simulink model "Test_FourMotor_PID_simcape_motor"  (R2025a)
settings: Solver=FixedStepAuto  StartTime=0.0  StopTime=2  FixedStep=50e-5  RelTol=1e-3
values from neighbouring files (symbols this model uses):
  Ki_id = 710.3004    [EMRAX348_DQData.m]    (also in Evolito_D500_DQData.m = 281.669634183)
  Ki_iq = 1.0615e3    (= 1061.5)    [EMRAX348_DQData.m]    (also in Evolito_D500_DQData.m = 420.937840785)
  Kp_id = 0.8779    [EMRAX348_DQData.m]    (also in Evolito_D500_DQData.m = 0.144107025607)
  Kp_iq = 1.0744    [EMRAX348_DQData.m]    (also in Evolito_D500_DQData.m = 0.144418307682)
  Ld = 52e-6    (= 5.2e-05)    [EMRAX348_DQData.m]    (also in Evolito_D500_DQData.m = 4e-05; pmsm_batt_testbench_data.m = 4e-05)
  Lq = 52e-6    (= 5.2e-05)    [EMRAX348_DQData.m]    (also in Evolito_D500_DQData.m = 4e-05; pmsm_batt_testbench_data.m = 4e-05)
  p = 10    [EMRAX348_DQData.m]    (also in Evolito_D500_DQData.m; pmsm_batt_testbench_data.m)
  psim = 0.06249    [EMRAX348_DQData.m]    (also in Evolito_D500_DQData.m = 0.045; pmsm_batt_testbench_data.m = 0.045)
undefined symbols (not defined in the file or in its folder): Limit, motorctrl, RPM
libraries: fl_lib x101, nesl_utility x37, eeDiscretePi x8, slpidlib x7, eeDqVoltageLimiter x4, eePmsmCurrentReferenceGen x4, eePmsmTorqueEstimator x4, ee_lib x4, batteryecm_lib x2, HEV_Battery_Lib x1, spspowerguiLib x1
(part 1 of 3)
settings Model: Creator=froshoo  LastModifiedBy=froshoo
settings DataIOCC: SaveOutput=off  SignalLogging=off  DSMLogging=off  SaveTime=off  ReturnWorkspaceOutputs=off
settings SimscapeCC: SimscapeLogType=all  SimscapeLogSimulationStatistics=on  SimscapeLogToSDI=on  SimscapeLogOpenViewer=on

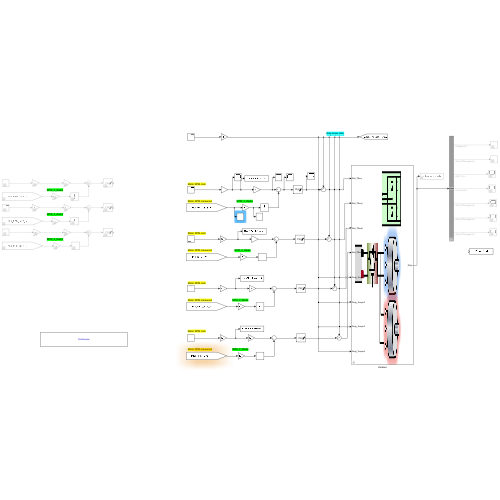
[thumbnail: Simulink's stored preview of the top-level diagram]
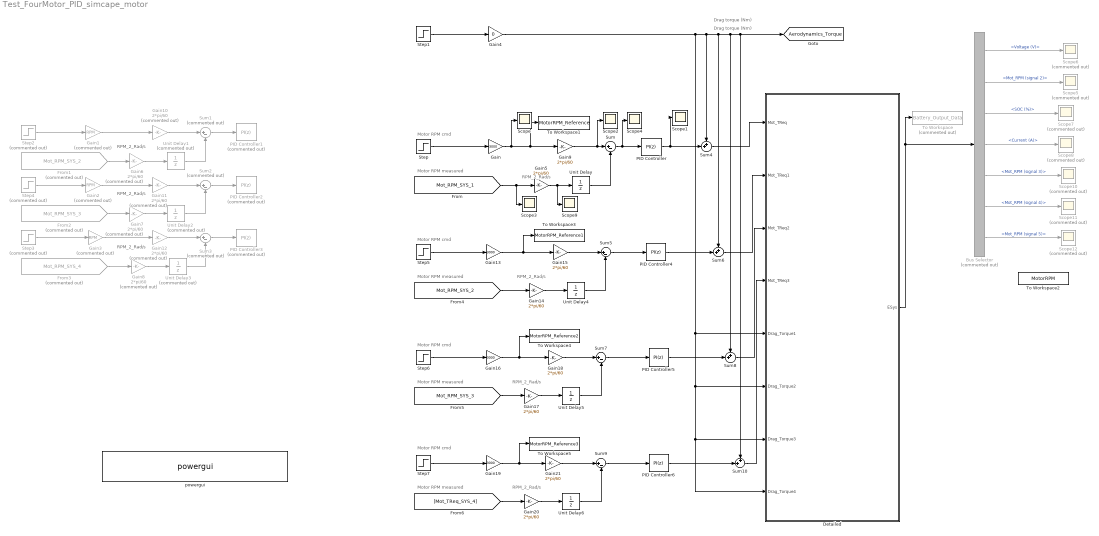
== system Test_FourMotor_PID_simcape_motor ==
  note: Motor RPM cmd
  note: Motor RPM measured
  note: RPM_2_Rad/s
  note: RPM_2_Rad/s
  note: RPM_2_Rad/s
  note: RPM_2_Rad/s
  note: Drag torque (Nm)
  note: Drag torque (Nm)
  note: RPM_2_Rad/s
  note: Motor RPM cmd
  note: Motor RPM measured
  note: Motor RPM measured
  note: RPM_2_Rad/s
  note: Motor RPM cmd
  note: Motor RPM cmd
  note: Motor RPM measured
  note: RPM_2_Rad/s
  Bus Selector : BusSelector  Commented=on  OutputSignals=Batt (signal 1).Voltage (V),Mot_RPM (signal 2),Batt (signal 1).SOC (%),Batt (signal 1).Current (A),Mot_RPM (signal 3),Mot_RPM (signal 4),Mot_RPM (signal 5)
  Detailed : Subsystem  mask{popup_batteryvariant=Cells}
      mask prompts: popup_batteryvariant "Battery Model"
      mask init:
      | set_param([gcb '/Battery'],'LabelModeActiveChoice',get_param(gcb,'popup_batteryvariant'));
      mask TypeOptions popup_batteryvariant: Predefined | Cells | Generic
      mask Display: image('HEV_Electrical_Detailed_IMAGE.jpg');
  From1 : From  Commented=on  GotoTag=Mot_RPM_SYS_2  TagVisibility=global
  From2 : From  Commented=on  GotoTag=Mot_RPM_SYS_3  TagVisibility=global
  From3 : From  Commented=on  GotoTag=Mot_RPM_SYS_4  TagVisibility=global
  Gain{,13,16,19} (4 alike) : Gain  Gain=3000
  Gain1 : Gain  Commented=on  Gain=RPM
  Gain{6..8,10..12} (6 alike) : Gain  Commented=on  Gain=2*pi/60
  Gain{5,9,14..15,17..18,20..21} (8 alike) : Gain  Gain=2*pi/60
  Gain2 : Gain  Commented=on  Gain=RPM
  Gain3 : Gain  Commented=on  Gain=RPM
  Gain4 : Gain  Gain=0
  PID Controller{,4..6} (4 alike) : slpidlib/PID Controller  Controller=PI  Form=Parallel  TimeDomain=Discrete-time  UseExternalTs=off  SampleTime=0.005  IntegratorMethod=Forward Euler  FilterMethod=Forward Euler  ControllerParametersSource=internal  P=0.4  I=0.5  UseKiTs=off  D=motorctrl.d  UseExternalDerivativeSource=off  N=motorctrl.n  UseFilter=on  TunerSelectOption=Transfer Function Based (PID Tuner App)  InitialConditionSource=internal  InitialConditionForIntegrator=0  InitialConditionForFilter=0  DifferentiatorICPrevScaledInput=0  ExternalReset=none  TrackingMode=off  Kt=1  LimitOutput=on  SatLimitsSource=internal  UpperSaturationLimit=800  LowerSaturationLimit=-800  LinearizeAsGain=on  AntiWindupMode=back-calculation  Kb=1  LimitIntegrator=off  UpperIntegratorSaturationLimit=inf  LowerIntegratorSaturationLimit=-inf  POutMin=[]  POutMax=[]  IOutMin=[]  IOutMax=[]  DOutMin=[]  DOutMax=[]  NOutMin=[]  NOutMax=[]  SumOutMin=[]  SumOutMax=[]  SaturationOutMin=[]  SaturationOutMax=[]  PParamMin=[]  PParamMax=[]  IParamMin=[]  IParamMax=[]  DParamMin=[]  DParamMax=[]  NParamMin=[]  NParamMax=[]  KbParamMin=[]  KbParamMax=[]  KtParamMin=[]  KtParamMax=[]  KbOutMin=[]  KbOutMax=[]  KtOutMin=[]  KtOutMax=[]  IntegratorOutMin=[]  IntegratorOutMax=[]  FilterOutMin=[]  FilterOutMax=[]  SumI1OutMin=[]  SumI1OutMax=[]  SumI2OutMin=[]  SumI2OutMax=[]  SumI3OutMin=[]  SumI3OutMax=[]  SumI4OutMin=[]  SumI4OutMax=[]  SumDOutMin=[]  SumDOutMax=[]  DifferentiatorOutMin=[]  DifferentiatorOutMax=[]  FilterDiffOutCoefMin=[]  FilterDiffOutCoefMax=[]  ReciprocalOutMin=[]  ReciprocalOutMax=[]  SumDenOutMin=[]  SumDenOutMax=[]  SumNumOutMin=[]  SumNumOutMax=[]  DivideOutMin=[]  DivideOutMax=[]  UdiffTsProdOutMin=[]  UdiffTsProdOutMax=[]  NTsProdOutMin=[]  NTsProdOutMax=[]  UintegralTsProdOutMin=[]  UintegralTsProdOutMax=[]  UngainTsProdOutMin=[]  UngainTsProdOutMax=[]  ClampingZeroOutDataTypeStr=Inherit: Inherit via back propagation  ClampingZeroOutMin=[]  ClampingZeroOutMax=[]  FilterDenConstantOutDataTypeStr=Inherit: Inherit via back propagation  FilterDenConstantOutMin=[]  FilterDenConstantOutMax=[]  PCopyOutDataTypeStr=Inherit: Inherit via back propagation  PCopyOutMin=[]  PCopyOutMax=[]  NCopyOutDataTypeStr=Inherit: Inherit via back propagation  NCopyOutMin=[]  NCopyOutMax=[]  IntegratorContinuousStateAttributes=''  IntegratorStateMustResolveToSignalObject=off  IntegratorRTWStateStorageClass=Auto  FilterContinuousStateAttributes=''  FilterStateMustResolveToSignalObject=off  FilterRTWStateStorageClass=Auto  ParallelPVariant=InternalParameters  IdealPVariant=Disabled  IVariant=InternalParameters  DVariant=Disabled  IntegratorVariant=Discrete  SatVariant=Enabled  AWVariant=BackCalculation  PCopyVariant=Disabled  TRVariant=Disabled  FdbkBlocksVariant=Forward  IdealPFdbkVariant=Disabled  SatFdbkVariant=Disabled  DerivativeFilterVariant=Disabled  NVariant=Disabled  NCopyVariant=Disabled_SignalSpec  FilterICVariant=Disabled  IntegratorICVariant=InternalICs  ExternalResetVariant=Disabled  TRSumVariant=Passthrough  SumFdbkVariant=Disabled  SumVariant=Sum_PI  TsampFilterVariant=InternalTs  TsampNgainVariant=Passthrough  TsampIntegralVariant=Disabled_SignalSpec  ExternalSaturationOutDataTypeStr=Inherit: Same as second input  DerivativeSourceVariant=Disabled  PreIntVariant=InternalPreInt
  PID Controller1 : slpidlib/PID Controller  Commented=on  Controller=PI  Form=Parallel  TimeDomain=Discrete-time  UseExternalTs=off  SampleTime=0.005  IntegratorMethod=Forward Euler  FilterMethod=Forward Euler  ControllerParametersSource=internal  P=motorctrl.p  I=motorctrl.i  UseKiTs=off  D=motorctrl.d  UseExternalDerivativeSource=off  N=motorctrl.n  UseFilter=on  TunerSelectOption=Transfer Function Based (PID Tuner App)  InitialConditionSource=internal  InitialConditionForIntegrator=0  InitialConditionForFilter=0  DifferentiatorICPrevScaledInput=0  ExternalReset=none  TrackingMode=off  Kt=1  LimitOutput=on  SatLimitsSource=internal  UpperSaturationLimit=Limit  LowerSaturationLimit=-Limit  LinearizeAsGain=on  AntiWindupMode=back-calculation  Kb=1  LimitIntegrator=off  UpperIntegratorSaturationLimit=inf  LowerIntegratorSaturationLimit=-inf  POutMin=[]  POutMax=[]  IOutMin=[]  IOutMax=[]  DOutMin=[]  DOutMax=[]  NOutMin=[]  NOutMax=[]  SumOutMin=[]  SumOutMax=[]  SaturationOutMin=[]  SaturationOutMax=[]  PParamMin=[]  PParamMax=[]  IParamMin=[]  IParamMax=[]  DParamMin=[]  DParamMax=[]  NParamMin=[]  NParamMax=[]  KbParamMin=[]  KbParamMax=[]  KtParamMin=[]  KtParamMax=[]  KbOutMin=[]  KbOutMax=[]  KtOutMin=[]  KtOutMax=[]  IntegratorOutMin=[]  IntegratorOutMax=[]  FilterOutMin=[]  FilterOutMax=[]  SumI1OutMin=[]  SumI1OutMax=[]  SumI2OutMin=[]  SumI2OutMax=[]  SumI3OutMin=[]  SumI3OutMax=[]  SumI4OutMin=[]  SumI4OutMax=[]  SumDOutMin=[]  SumDOutMax=[]  DifferentiatorOutMin=[]  DifferentiatorOutMax=[]  FilterDiffOutCoefMin=[]  FilterDiffOutCoefMax=[]  ReciprocalOutMin=[]  ReciprocalOutMax=[]  SumDenOutMin=[]  SumDenOutMax=[]  SumNumOutMin=[]  SumNumOutMax=[]  DivideOutMin=[]  DivideOutMax=[]  UdiffTsProdOutMin=[]  UdiffTsProdOutMax=[]  NTsProdOutMin=[]  NTsProdOutMax=[]  UintegralTsProdOutMin=[]  UintegralTsProdOutMax=[]  UngainTsProdOutMin=[]  UngainTsProdOutMax=[]  ClampingZeroOutDataTypeStr=Inherit: Inherit via back propagation  ClampingZeroOutMin=[]  ClampingZeroOutMax=[]  FilterDenConstantOutDataTypeStr=Inherit: Inherit via back propagation  FilterDenConstantOutMin=[]  FilterDenConstantOutMax=[]  PCopyOutDataTypeStr=Inherit: Inherit via back propagation  PCopyOutMin=[]  PCopyOutMax=[]  NCopyOutDataTypeStr=Inherit: Inherit via back propagation  NCopyOutMin=[]  NCopyOutMax=[]  IntegratorContinuousStateAttributes=''  IntegratorStateMustResolveToSignalObject=off  IntegratorRTWStateStorageClass=Auto  FilterContinuousStateAttributes=''  FilterStateMustResolveToSignalObject=off  FilterRTWStateStorageClass=Auto  ParallelPVariant=InternalParameters  IdealPVariant=Disabled  IVariant=InternalParameters  DVariant=Disabled  IntegratorVariant=Discrete  SatVariant=Enabled  AWVariant=BackCalculation  PCopyVariant=Disabled  TRVariant=Disabled  FdbkBlocksVariant=Forward  IdealPFdbkVariant=Disabled  SatFdbkVariant=Disabled  DerivativeFilterVariant=Disabled  NVariant=Disabled  NCopyVariant=Disabled_SignalSpec  FilterICVariant=Disabled  IntegratorICVariant=InternalICs  ExternalResetVariant=Disabled  TRSumVariant=Passthrough  SumFdbkVariant=Disabled  SumVariant=Sum_PI  TsampFilterVariant=InternalTs  TsampNgainVariant=Passthrough  TsampIntegralVariant=Disabled_SignalSpec  ExternalSaturationOutDataTypeStr=Inherit: Same as second input  DerivativeSourceVariant=Disabled  PreIntVariant=InternalPreInt
  PID Controller2 : slpidlib/PID Controller  Commented=on  Controller=PI  Form=Parallel  TimeDomain=Discrete-time  UseExternalTs=off  SampleTime=0.005  IntegratorMethod=Forward Euler  FilterMethod=Forward Euler  ControllerParametersSource=internal  P=motorctrl.p  I=motorctrl.i  UseKiTs=off  D=motorctrl.d  UseExternalDerivativeSource=off  N=motorctrl.n  UseFilter=on  TunerSelectOption=Transfer Function Based (PID Tuner App)  InitialConditionSource=internal  InitialConditionForIntegrator=0  InitialConditionForFilter=0  DifferentiatorICPrevScaledInput=0  ExternalReset=none  TrackingMode=off  Kt=1  LimitOutput=on  SatLimitsSource=internal  UpperSaturationLimit=Limit  LowerSaturationLimit=-Limit  LinearizeAsGain=on  AntiWindupMode=back-calculation  Kb=1  LimitIntegrator=off  UpperIntegratorSaturationLimit=inf  LowerIntegratorSaturationLimit=-inf  POutMin=[]  POutMax=[]  IOutMin=[]  IOutMax=[]  DOutMin=[]  DOutMax=[]  NOutMin=[]  NOutMax=[]  SumOutMin=[]  SumOutMax=[]  SaturationOutMin=[]  SaturationOutMax=[]  PParamMin=[]  PParamMax=[]  IParamMin=[]  IParamMax=[]  DParamMin=[]  DParamMax=[]  NParamMin=[]  NParamMax=[]  KbParamMin=[]  KbParamMax=[]  KtParamMin=[]  KtParamMax=[]  KbOutMin=[]  KbOutMax=[]  KtOutMin=[]  KtOutMax=[]  IntegratorOutMin=[]  IntegratorOutMax=[]  FilterOutMin=[]  FilterOutMax=[]  SumI1OutMin=[]  SumI1OutMax=[]  SumI2OutMin=[]  SumI2OutMax=[]  SumI3OutMin=[]  SumI3OutMax=[]  SumI4OutMin=[]  SumI4OutMax=[]  SumDOutMin=[]  SumDOutMax=[]  DifferentiatorOutMin=[]  DifferentiatorOutMax=[]  FilterDiffOutCoefMin=[]  FilterDiffOutCoefMax=[]  ReciprocalOutMin=[]  ReciprocalOutMax=[]  SumDenOutMin=[]  SumDenOutMax=[]  SumNumOutMin=[]  SumNumOutMax=[]  DivideOutMin=[]  DivideOutMax=[]  UdiffTsProdOutMin=[]  UdiffTsProdOutMax=[]  NTsProdOutMin=[]  NTsProdOutMax=[]  UintegralTsProdOutMin=[]  UintegralTsProdOutMax=[]  UngainTsProdOutMin=[]  UngainTsProdOutMax=[]  ClampingZeroOutDataTypeStr=Inherit: Inherit via back propagation  ClampingZeroOutMin=[]  ClampingZeroOutMax=[]  FilterDenConstantOutDataTypeStr=Inherit: Inherit via back propagation  FilterDenConstantOutMin=[]  FilterDenConstantOutMax=[]  PCopyOutDataTypeStr=Inherit: Inherit via back propagation  PCopyOutMin=[]  PCopyOutMax=[]  NCopyOutDataTypeStr=Inherit: Inherit via back propagation  NCopyOutMin=[]  NCopyOutMax=[]  IntegratorContinuousStateAttributes=''  IntegratorStateMustResolveToSignalObject=off  IntegratorRTWStateStorageClass=Auto  FilterContinuousStateAttributes=''  FilterStateMustResolveToSignalObject=off  FilterRTWStateStorageClass=Auto  ParallelPVariant=InternalParameters  IdealPVariant=Disabled  IVariant=InternalParameters  DVariant=Disabled  IntegratorVariant=Discrete  SatVariant=Enabled  AWVariant=BackCalculation  PCopyVariant=Disabled  TRVariant=Disabled  FdbkBlocksVariant=Forward  IdealPFdbkVariant=Disabled  SatFdbkVariant=Disabled  DerivativeFilterVariant=Disabled  NVariant=Disabled  NCopyVariant=Disabled_SignalSpec  FilterICVariant=Disabled  IntegratorICVariant=InternalICs  ExternalResetVariant=Disabled  TRSumVariant=Passthrough  SumFdbkVariant=Disabled  SumVariant=Sum_PI  TsampFilterVariant=InternalTs  TsampNgainVariant=Passthrough  TsampIntegralVariant=Disabled_SignalSpec  ExternalSaturationOutDataTypeStr=Inherit: Same as second input  DerivativeSourceVariant=Disabled  PreIntVariant=InternalPreInt
  PID Controller3 : slpidlib/PID Controller  Commented=on  Controller=PI  Form=Parallel  TimeDomain=Discrete-time  UseExternalTs=off  SampleTime=0.005  IntegratorMethod=Forward Euler  FilterMethod=Forward Euler  ControllerParametersSource=internal  P=motorctrl.p  I=motorctrl.i  UseKiTs=off  D=motorctrl.d  UseExternalDerivativeSource=off  N=motorctrl.n  UseFilter=on  TunerSelectOption=Transfer Function Based (PID Tuner App)  InitialConditionSource=internal  InitialConditionForIntegrator=0  InitialConditionForFilter=0  DifferentiatorICPrevScaledInput=0  ExternalReset=none  TrackingMode=off  Kt=1  LimitOutput=on  SatLimitsSource=internal  UpperSaturationLimit=Limit  LowerSaturationLimit=-Limit  LinearizeAsGain=on  AntiWindupMode=back-calculation  Kb=1  LimitIntegrator=off  UpperIntegratorSaturationLimit=inf  LowerIntegratorSaturationLimit=-inf  POutMin=[]  POutMax=[]  IOutMin=[]  IOutMax=[]  DOutMin=[]  DOutMax=[]  NOutMin=[]  NOutMax=[]  SumOutMin=[]  SumOutMax=[]  SaturationOutMin=[]  SaturationOutMax=[]  PParamMin=[]  PParamMax=[]  IParamMin=[]  IParamMax=[]  DParamMin=[]  DParamMax=[]  NParamMin=[]  NParamMax=[]  KbParamMin=[]  KbParamMax=[]  KtParamMin=[]  KtParamMax=[]  KbOutMin=[]  KbOutMax=[]  KtOutMin=[]  KtOutMax=[]  IntegratorOutMin=[]  IntegratorOutMax=[]  FilterOutMin=[]  FilterOutMax=[]  SumI1OutMin=[]  SumI1OutMax=[]  SumI2OutMin=[]  SumI2OutMax=[]  SumI3OutMin=[]  SumI3OutMax=[]  SumI4OutMin=[]  SumI4OutMax=[]  SumDOutMin=[]  SumDOutMax=[]  DifferentiatorOutMin=[]  DifferentiatorOutMax=[]  FilterDiffOutCoefMin=[]  FilterDiffOutCoefMax=[]  ReciprocalOutMin=[]  ReciprocalOutMax=[]  SumDenOutMin=[]  SumDenOutMax=[]  SumNumOutMin=[]  SumNumOutMax=[]  DivideOutMin=[]  DivideOutMax=[]  UdiffTsProdOutMin=[]  UdiffTsProdOutMax=[]  NTsProdOutMin=[]  NTsProdOutMax=[]  UintegralTsProdOutMin=[]  UintegralTsProdOutMax=[]  UngainTsProdOutMin=[]  UngainTsProdOutMax=[]  ClampingZeroOutDataTypeStr=Inherit: Inherit via back propagation  ClampingZeroOutMin=[]  ClampingZeroOutMax=[]  FilterDenConstantOutDataTypeStr=Inherit: Inherit via back propagation  FilterDenConstantOutMin=[]  FilterDenConstantOutMax=[]  PCopyOutDataTypeStr=Inherit: Inherit via back propagation  PCopyOutMin=[]  PCopyOutMax=[]  NCopyOutDataTypeStr=Inherit: Inherit via back propagation  NCopyOutMin=[]  NCopyOutMax=[]  IntegratorContinuousStateAttributes=''  IntegratorStateMustResolveToSignalObject=off  IntegratorRTWStateStorageClass=Auto  FilterContinuousStateAttributes=''  FilterStateMustResolveToSignalObject=off  FilterRTWStateStorageClass=Auto  ParallelPVariant=InternalParameters  IdealPVariant=Disabled  IVariant=InternalParameters  DVariant=Disabled  IntegratorVariant=Discrete  SatVariant=Enabled  AWVariant=BackCalculation  PCopyVariant=Disabled  TRVariant=Disabled  FdbkBlocksVariant=Forward  IdealPFdbkVariant=Disabled  SatFdbkVariant=Disabled  DerivativeFilterVariant=Disabled  NVariant=Disabled  NCopyVariant=Disabled_SignalSpec  FilterICVariant=Disabled  IntegratorICVariant=InternalICs  ExternalResetVariant=Disabled  TRSumVariant=Passthrough  SumFdbkVariant=Disabled  SumVariant=Sum_PI  TsampFilterVariant=InternalTs  TsampNgainVariant=Passthrough  TsampIntegralVariant=Disabled_SignalSpec  ExternalSaturationOutDataTypeStr=Inherit: Same as second input  DerivativeSourceVariant=Disabled  PreIntVariant=InternalPreInt
  Scope{,1..4,9} (6 alike) : Scope
      Scope settings: ActiveDisplayYMinimum=2000  ActiveDisplayYMaximum=4000
      Scope1 settings: ActiveDisplayYMinimum=-481.89960137193771  ActiveDisplayYMaximum=332.79708047153025
      Scope2 settings: ActiveDisplayYMinimum=214.15926535897933  ActiveDisplayYMaximum=414.15926535897933  DataLoggingVariableName=ScopeData17
      Scope3 settings: ActiveDisplayYMinimum=-443.57556490404767  ActiveDisplayYMaximum=3992.18008413643  DataLoggingVariableName=ScopeData19
      Scope4 settings: ActiveDisplayYMinimum=-39.421537573321494  ActiveDisplayYMaximum=353.44602124034606  DataLoggingVariableName=ScopeData20
      Scope9 settings: ActiveDisplayYMinimum=-46.359271320847974  ActiveDisplayYMaximum=417.23344188763184  DataLoggingVariableName=ScopeData21
  Scope{5..8,10..12} (7 alike) : Scope  Commented=on
      Scope10 settings: ActiveDisplayYMinimum=-838.99189969639019  ActiveDisplayYMaximum=7550.927097267514  DataLoggingVariableName=ScopeData18
      Scope11 settings: ActiveDisplayYMinimum=-838.99189969639019  ActiveDisplayYMaximum=7550.927097267514  DataLoggingVariableName=ScopeData22
      Scope12 settings: ActiveDisplayYMinimum=-838.99189969639019  ActiveDisplayYMaximum=7550.927097267514  DataLoggingVariableName=ScopeData23
      Scope5 settings: ActiveDisplayYMinimum=-838.99189969639019  ActiveDisplayYMaximum=7550.927097267514  DataLoggingVariableName=ScopeData2
      Scope6 settings: ActiveDisplayYMinimum=813.40102643578655  ActiveDisplayYMaximum=813.74696487540177  DataLoggingVariableName=ScopeData3
      Scope7 settings: ActiveDisplayYMinimum=99.00226  ActiveDisplayYMaximum=100.11086  DataLoggingVariableName=ScopeData4
      Scope8 settings: ActiveDisplayYMinimum=-1508.9225284750978  ActiveDisplayYMaximum=1817.2458957057474  DataLoggingVariableName=ScopeData5
  Step{,1,5..7} (5 alike) : Step  Time=0  SampleTime=0
  Step2 : Step  Commented=on  Time=0  SampleTime=0
  Step3 : Step  Commented=on  Time=0  SampleTime=0
  Step4 : Step  Commented=on  Time=0  SampleTime=0
  Sum{,5,7,9} (4 alike) : Sum  Inputs=|+-
  Sum1 : Sum  Commented=on  Inputs=|+-
  Sum{4,6,8,10} (4 alike) : Sum  Inputs=++|
  Sum2 : Sum  Commented=on  Inputs=|+-
  Sum3 : Sum  Commented=on  Inputs=|+-
  To Workspace : ToWorkspace  Commented=on  VariableName=Battery_Output_Data  SaveFormat=Timeseries  SampleTime=-1
  To Workspace1 : ToWorkspace  VariableName=MotorRPM_Reference  SaveFormat=Timeseries  SampleTime=-1
  To Workspace2 : ToWorkspace  VariableName=MotorRPM  SaveFormat=Timeseries  SampleTime=-1
  To Workspace3 : ToWorkspace  VariableName=MotorRPM_Reference1  SaveFormat=Timeseries  SampleTime=-1
  To Workspace4 : ToWorkspace  VariableName=MotorRPM_Reference2  SaveFormat=Timeseries  SampleTime=-1
  To Workspace5 : ToWorkspace  VariableName=MotorRPM_Reference3  SaveFormat=Timeseries  SampleTime=-1
  Unit Delay{,4..6} (4 alike) : UnitDelay  SampleTime=-1  HasFrameUpgradeWarning=on
  Unit Delay1 : UnitDelay  Commented=on  SampleTime=-1  HasFrameUpgradeWarning=on
  Unit Delay2 : UnitDelay  Commented=on  SampleTime=-1  HasFrameUpgradeWarning=on
  Unit Delay3 : UnitDelay  Commented=on  SampleTime=-1  HasFrameUpgradeWarning=on
  powergui : spspowerguiLib/powergui  Priority=1  SimulationMode=Continuous  SampleTime=50e-6  frequency=60  Iterations=50  frequencyindice=0  Pbase=100e6  ErrMax=1e-4  UnitsV=kV  UnitsW=MW  buscounter=0  FunctionMessages=off  echomessages=off  EnableUseOfTLC=off  CurrentSourceSwitches=off  DisableSnubberDevices=off  DisableRonSwitches=off  DisableVfSwitches=off  DisplayEquations=off  AutomaticDiscreteSolvers=off  SolverType=Tustin/Backward Euler (TBE)  Interpol=off  ExternalGateDelay=off  methode=off  Ts=100  x0status=blocks  SPID=on  SwTol=0  HookPort=off  NonlinearTolerance=1e-4  nMaxIteration=100  ContinueOnMaxIteration=off  RestoreLinks=warning  ResistiveCurrentMeasurement=off  Frange=[0:2:500]  Ylog=off  Xlog=on  ShowGrid=off  save=off  variable=ZData  structure=0  ZoomFFT=off  StartTime=0.0  cycles=1  DisplayStyle=1  fundamental=60  FreqAxis=off  MaxFrequency=1000  frequencyindicesteady=1  RmsSteady=1  display=off
  tag scope: Aerodynamics_Torque=global
  wires:
  Sum/1 -> Scope4/1, PID Controller/1
  From1/1 -> Gain6/1
  Sum1/1 -> PID Controller1/1
  Sum2/1 -> PID Controller2/1
  From3/1 -> Gain8/1
  Sum3/1 -> PID Controller3/1
  Detailed/1(ESys) -> To Workspace/1, Bus Selector/1
  Step/1 -> Gain/1
  Step3/1 -> Gain3/1
  Step4/1 -> Gain2/1
  Step2/1 -> Gain1/1
  Gain/1 -> To Workspace1/1, Gain9/1, Scope/1
  Gain1/1 -> Gain10/1
  Gain2/1 -> Gain11/1
  Gain3/1 -> Gain12/1
  [Mot_RPM_SYS_1] -> Gain5/1, Scope3/1
  Unit Delay/1 -> Sum/2
  Unit Delay1/1 -> Sum1/2
  Unit Delay2/1 -> Sum2/2
  Unit Delay3/1 -> Sum3/2
  From2/1 -> Gain7/1
  Step1/1 -> Gain4/1
  Gain5/1 -> Scope9/1, Unit Delay/1
  Gain6/1 -> Unit Delay1/1
  Gain7/1 -> Unit Delay2/1
  Gain8/1 -> Unit Delay3/1
  Gain9/1 -> Scope2/1, Sum/1
  Gain10/1 -> Sum1/1
  Gain11/1 -> Sum2/1
  Gain12/1 -> Sum3/1
  PID Controller/1 -> Sum4/2, Scope1/1
  Sum4/1 -> Detailed/1(Mot_TReq)
  PID Controller4/1 -> Sum6/2
  Gain15/1 -> Sum5/1
  Sum5/1 -> PID Controller4/1
  [Mot_RPM_SYS_2] -> Gain14/1
  Sum6/1 -> Detailed/2(Mot_TReq1)
  Step5/1 -> Gain13/1
  Gain14/1 -> Unit Delay4/1
  Unit Delay4/1 -> Sum5/2
  Gain13/1 -> To Workspace3/1, Gain15/1
  Sum7/1 -> PID Controller5/1
  Gain18/1 -> Sum7/1
  PID Controller5/1 -> Sum8/2
  Gain17/1 -> Unit Delay5/1
  Step6/1 -> Gain16/1
  Gain16/1 -> To Workspace4/1, Gain18/1
  Sum8/1 -> Detailed/3(Mot_TReq2)
  [Mot_RPM_SYS_3] -> Gain17/1
  Unit Delay5/1 -> Sum7/2
  Unit Delay6/1 -> Sum9/2
  Gain21/1 -> Sum9/1
  Sum10/1 -> Detailed/4(Mot_TReq3)
  Step7/1 -> Gain19/1
  PID Controller6/1 -> Sum10/2
  Sum9/1 -> PID Controller6/1
  Gain19/1 -> To Workspace5/1, Gain21/1
  Gain20/1 -> Unit Delay6/1
  [Mot_TReq_SYS_4] -> Gain20/1
  Gain4/1 -> Detailed/5(Drag_Torque1), Detailed/6(Drag_Torque2), Detailed/7(Drag_Torque3), Detailed/8(Drag_Torque4), [Aerodynamics_Torque], Sum10/1, Sum8/1, Sum6/1, Sum4/1
  Bus Selector/1 -> Scope6/1  "<Voltage (V)>"
  Bus Selector/2 -> Scope5/1  "<Mot_RPM (signal 2)>"
  Bus Selector/3 -> Scope7/1  "<SOC (%)>"
  Bus Selector/4 -> Scope8/1  "<Current (A)>"
  Bus Selector/5 -> Scope10/1  "<Mot_RPM (signal 3)>"
  Bus Selector/6 -> Scope11/1  "<Mot_RPM (signal 4)>"
  Bus Selector/7 -> Scope12/1  "<Mot_RPM (signal 5)>"

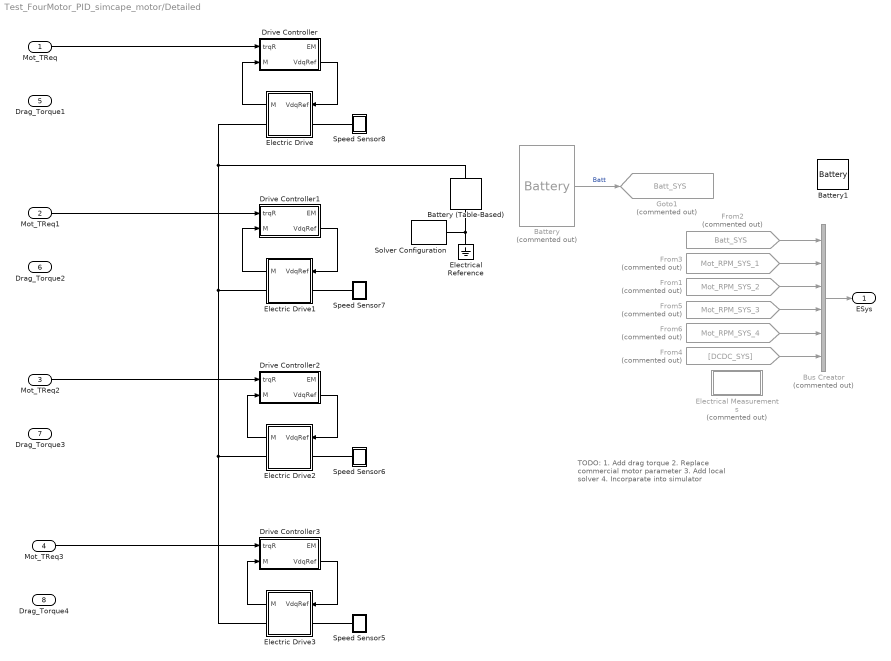
== system Test_FourMotor_PID_simcape_motor/Detailed ==
  note: TODO:
      | 1.  Add drag torque
      | 2. Replace commercial motor parameter
      | 3. Add local solver
      | 4. Incorparate into simulator
  Mot_TReq : Inport
  Mot_TReq1 : Inport  Port=2
  Mot_TReq2 : Inport  Port=3
  Mot_TReq3 : Inport  Port=4
  Drag_Torque1 : Inport  Port=5
  Drag_Torque2 : Inport  Port=6
  Drag_Torque3 : Inport  Port=7
  Drag_Torque4 : Inport  Port=8
  Battery : HEV_Battery_Lib/Battery  Commented=on  SystemSampleTime=-1  LabelModeActiveChoice=Cells  VariantActivationTime=update diagram  EmptyChoice=off  PassThrough=off  PassThroughVariantControl=(default)  EmptyChoiceVariantControl=(default)  AllowFlexibleInterface=on  Latency=0  AutoFrameSizeCalculation=off
  Battery (Table-Based) : batteryecm_lib/Battery (Table-Based)  SOC_vec=HEV_Param.Battery_Cell.SOC  T_dependence=simscape.enum.tablebattery.temperature_dependence.no  prm_dir=simscape.enum.tablebattery.prm_dir.noCurrentDirectionality  T_vec=[297] K  V0_mat=HEV_Param.Battery_Cell.Emo V  V0_vec=HEV_Param.Battery_Cell.Emo V  V_range=[0, inf] V  R0_mat=HEV_Param.Battery_Cell.R0 Ohm  R0_vec=HEV_Param.Battery_Cell.R0 Ohm  R0_dis_mat=[.0117, .0085, .009; .011, .0085, .009; .0114, .0087, .0092; .0107, .0082, .0088; .0107, .0083, .0091; .0113, .0085, .0089; .0116, .0085, .0089] Ohm  R0_dis_vec=[.0085, .0085, .0087, .0082, .0083, .0085, .0085] Ohm  R0_ch_mat=[.0117, .0085, .009; .011, .0085, .009; .0114, .0087, .0092; .0107, .0082, .0088; .0107, .0083, .0091; .0113, .0085, .0089; .0116, .0085, .0089] Ohm  R0_ch_vec=[.0085, .0085, .0087, .0082, .0083, .0085, .0085] Ohm  AH=HEV_Param.Battery_Pack_Capacity Ah  prm_leak=simscape.enum.tablebattery.prm_leak.disabled  Rleak_vec=[8000, 7000, 6000] Ohm  Rleak=7e3 Ohm  extrapolation_option=simscape.enum.extrapolation.nearest  SOC_port=simscape.enum.tablebattery.enable.no  prm_dyn=simscape.enum.tablebattery.prm_dyn.rc1  R1_mat=HEV_Param.Battery_Cell.R1 Ohm  R1_vec=HEV_Param.Battery_Cell.R1 Ohm  tau1_mat=HEV_Param.Battery_Cell.Tau1 s  tau1_vec=HEV_Param.Battery_Cell.Tau1 s  R2_mat=HEV_Param.Battery_Cell.R2 Ohm  R2_vec=HEV_Param.Battery_Cell.R2 Ohm  tau2_mat=HEV_Param.Battery_Cell.Tau2 s  tau2_vec=HEV_Param.Battery_Cell.Tau2 s  R3_mat=[.0109, .0029, .0013; .0069, .0024, .0012; .0047, .0026, .0013; .0034, .0016, .001; .0033, .0023, .0014; .0033, .0018, .0011; .0028, .0017, .0011] Ohm  R3_vec=[.0029, .0024, .0026, .0016, .0023, .0018, .0017] Ohm  tau3_mat=[20, 36, 39; 31, 45, 39; 109, 105, 61; 36, 29, 26; 59, 77, 67; 40, 33, 29; 25, 39, 33] s  tau3_vec=[36, 45, 105, 29, 77, 33, 39] s  R4_mat=[.0109, .0029, .0013; .0069, .0024, .0012; .0047, .0026, .0013; .0034, .0016, .001; .0033, .0023, .0014; .0033, .0018, .0011; .0028, .0017, .0011] Ohm  R4_vec=[.0029, .0024, .0026, .0016, .0023, .0018, .0017] Ohm  tau4_mat=[20, 36, 39; 31, 45, 39; 109, 105, 61; 36, 29, 26; 59, 77, 67; 40, 33, 29; 25, 39, 33] s  tau4_vec=[36, 45, 105, 29, 77, 33, 39] s  R5_mat=[.0109, .0029, .0013; .0069, .0024, .0012; .0047, .0026, .0013; .0034, .0016, .001; .0033, .0023, .0014; .0033, .0018, .0011; .0028, .0017, .0011] Ohm  R5_vec=[.0029, .0024, .0026, .0016, .0023, .0018, .0017] Ohm  tau5_mat=[20, 36, 39; 31, 45, 39; 109, 105, 61; 36, 29, 26; 59, 77, 67; 40, 33, 29; 25, 39, 33] s  tau5_vec=[36, 45, 105, 29, 77, 33, 39] s  prm_fade=simscape.enum.tablebattery.prm_fade.disabled  N0=100  dV0=0  dR0=0  dAH=0  dRleak=0  dR1=0  dR2=0  dR3=0  dR4=0  dR5=0  N0vec=[0, 100, 200, 300]  Tfadevec=[298.15, 323.15] K  dV0vec=[0, 0, 0, 0]  dR0vec=[0, 0, 0, 0]  dAHvec=[0, 0, 0, 0]  dRleakvec=[0, 0, 0, 0]  dR1vec=[0, 0, 0, 0]  dR2vec=[0, 0, 0, 0]  dR3vec=[0, 0, 0, 0]  dR4vec=[0, 0, 0, 0]  dR5vec=[0, 0, 0, 0]  dV0mat=[0, 0; 0, 0; 0, 0; 0, 0]  dR0mat=[0, 0; 0, 0; 0, 0; 0, 0]  dAHmat=[0, 0; 0, 0; 0, 0; 0, 0]  dRleakmat=[0, 0; 0, 0; 0, 0; 0, 0]  dR1mat=[0, 0; 0, 0; 0, 0; 0, 0]  dR2mat=[0, 0; 0, 0; 0, 0; 0, 0]  dR3mat=[0, 0; 0, 0; 0, 0; 0, 0]  dR4mat=[0, 0; 0, 0; 0, 0; 0, 0]  dR5mat=[0, 0; 0, 0; 0, 0; 0, 0]  prm_age_modeling=simscape.enum.tablebattery.prm_age_modeling.equation  storage_dt_age_vec=[0] d  storage_T_age_vec=[273] K  prm_age_OCV=simscape.enum.tablebattery.prm_age_OCV.OCV  OCV_age=0.9  SOC_age=0.6  prm_age_resistance=simscape.enum.tablebattery.prm_age.disabled  OCV_scaling_age_resistance=2.2134e6  OCV_offset_age_resistance=1.632e6  temp_exp_age_resistance=0.515833569 V  t_exp_age_resistance=0.75  T_age_vec_resistance=[273.15, 298.15, 323.15] K  dt_age_vec_resistance=[0, 90, 180, 270] d  dR0_age_vec=[0, 0, 0]  t_meas_dR0_age=100 d  dR0_age_mat=[0, 0, 0; 0, 0, 0; 0, 0, 0; 0, 0, 0]  prm_age_capacity=simscape.enum.tablebattery.prm_age.disabled  OCV_scaling_age_capacity=1.5097e07  OCV_offset_age_capacity=8.3625e06  temp_exp_age_capacity=0.6011 V  t_exp_age_capacity=0.75  T_age_vec_capacity=[273.15, 298.15, 323.15] K  dt_age_vec_capacity=[0, 90, 180, 270] d  dAH_age_vec=[0, 0, 0]  t_meas_dAH_age=100 d  dAH_age_mat=[0, 0, 0; 0, 0, 0; 0, 0, 0; 0, 0, 0]  thermal_port=simscape.enum.thermaleffects.omit  temperature=298.15 K  thermal_mass=100 J/K  i_specify=off  i_priority=None  i=0 A  i_nominal_specify=off  i_nominal_value=1  i_nominal_unit=A  v_specify=off  v_priority=None  v=0 V  v_nominal_specify=off  v_nominal_value=1  v_nominal_unit=V  stateOfCharge_specify=off  stateOfCharge_priority=High  stateOfCharge=1  stateOfCharge_nominal_specify=off  stateOfCharge_nominal_value=1  stateOfCharge_nominal_unit=1  num_cycles_specify=off  num_cycles_priority=High  num_cycles=0  num_cycles_nominal_specify=off  num_cycles_nominal_value=1  num_cycles_nominal_unit=1  cell_temperature_specify=off  cell_temperature_priority=High  cell_temperature=298.15 K  cell_temperature_nominal_specify=off  cell_temperature_nominal_value=1  cell_temperature_nominal_unit=K
      settings: InternalSimscapePortConfiguration="{\"Bottom\":[],\"Left\":[{\"id\":\"p\",\"label\":\"+\",\"type\":\"foundation.electrical.electrical\"}],\"Right\":[{\"id\":\"n\",\"label\":\"-\",\"type\":\"foundation.electrical.electrical\"}],\"Top\":[]}"
  Battery1 : batteryecm_lib/Battery  Vnom=Vnom V  prm_dir=1  R1_dis=2 Ohm  R1_ch=2 Ohm  R1=0.001 Ohm  prm_AH=1  AH=300 hr*A  V1=V1 V  AH1=100 hr*A  prm_R2=1  R2=2000 Ohm  Tmeas=298.15 K  charge_measurement_port=simscape.enum.battery.enable.no  prm_dyn=simscape.enum.battery.prm_dyn.off  Rp1=0.005 Ohm  tau1=30 s  Rp2=0.005 Ohm  tau2=30 s  Rp3=0.005 Ohm  tau3=30 s  Rp4=0.005 Ohm  tau4=30 s  Rp5=0.005 Ohm  tau5=30 s  prm_fade=1  N_fade=100  AH_fade=45 hr*A  R1_fade=2.02 Ohm  R1_ch_fade=2.02 Ohm  V1_fade=10.35 V  prm_age=1  prm_age_OCV=1  OCV_age=0.9  SOC_age=60  Tmeas_age=298.15 K  delta_time_age_vec=[0] d  temperature_age_vec=[273] K  OCV_scaling_age=2.2134e6  OCV_offset_age=1.632e6  temp_exp_age=0.515833569 V  t_exp_age=0.75  Vnom_T2=12 V  R1_T2=2.2 Ohm  R1_T2_dis=2.2 Ohm  R1_T2_ch=2.2 Ohm  V1_T2=11.4 V  R2_T2=2200 Ohm  Rp1_T2=0.005 Ohm  tau1_T2=30 s  Rp2_T2=0.005 Ohm  tau2_T2=30 s  Rp3_T2=0.005 Ohm  tau3_T2=30 s  Rp4_T2=0.005 Ohm  tau4_T2=30 s  Rp5_T2=0.005 Ohm  tau5_T2=30 s  Tmeas2=273.15 K  thermal_port=simscape.enum.thermaleffects.omit  thermal_mass=30000 J/K  i_specify=off  i_priority=None  i=0 A  i_nominal_specify=off  i_nominal_value=1  i_nominal_unit=A  v_specify=off  v_priority=None  v=0 V  v_nominal_specify=off  v_nominal_value=1  v_nominal_unit=V  charge_specify=on  charge_priority=High  charge=AH0 hr*A  charge_nominal_specify=off  charge_nominal_value=1  charge_nominal_unit=A*hr  num_cycles_specify=off  num_cycles_priority=High  num_cycles=0  num_cycles_nominal_specify=off  num_cycles_nominal_value=1  num_cycles_nominal_unit=1  temperature_specify=off  temperature_priority=High  temperature=298.15 K  temperature_nominal_specify=off  temperature_nominal_value=1  temperature_nominal_unit=K
  Bus Creator : BusCreator  Commented=on  Inputs=6
  Drive Controller : Subsystem
  Drive Controller1 : Subsystem
  Drive Controller2 : Subsystem
  Drive Controller3 : Subsystem
  Electric Drive : Subsystem  Tag=PublishSubsystem
      mask Display:
      | % Circle
      | plot(sin(0:0.1:2.2*pi)*0.9,cos(0:0.1:2.2*pi)*0.9);
      | 
      | % In/out
      | plot([-1.1 -0.9],[0 0]);
      | plot([1.1 0.9],[0 0]);
      | 
      | % 'M'
      | plot([0.5 0.5],[-0.5 0.5]);
      | plot([-0.5 -0.5],[-0.5 0.5]);
      | plot([0.5 0],[0.5 -0.5]);
      | plot([-0.5 0],[0.5 -0.5]);
      | 
      | % Inputs and Outputs
      | plot([0.5 0.5],[0.9 1.8]);
      | plot([0.5 1.1],[1.8 1.8]);
      | 
      | plot([-0.5 -0.5],[0.9 1.8]);
      | plot([-0.5 -1.1],[1.8 1.8]);
      | 
      | 
      | % Plot points to set plot range
      | color('white');plot(1.9,2.8);plot(-1.9,0)
      | color('black');
  Electric Drive1 : Subsystem  Tag=PublishSubsystem
      mask Display:
      | % Circle
      | plot(sin(0:0.1:2.2*pi)*0.9,cos(0:0.1:2.2*pi)*0.9);
      | 
      | % In/out
      | plot([-1.1 -0.9],[0 0]);
      | plot([1.1 0.9],[0 0]);
      | 
      | % 'M'
      | plot([0.5 0.5],[-0.5 0.5]);
      | plot([-0.5 -0.5],[-0.5 0.5]);
      | plot([0.5 0],[0.5 -0.5]);
      | plot([-0.5 0],[0.5 -0.5]);
      | 
      | % Inputs and Outputs
      | plot([0.5 0.5],[0.9 1.8]);
      | plot([0.5 1.1],[1.8 1.8]);
      | 
      | plot([-0.5 -0.5],[0.9 1.8]);
      | plot([-0.5 -1.1],[1.8 1.8]);
      | 
      | 
      | % Plot points to set plot range
      | color('white');plot(1.9,2.8);plot(-1.9,0)
      | color('black');
  Electric Drive2 : Subsystem  Tag=PublishSubsystem
      mask Display:
      | % Circle
      | plot(sin(0:0.1:2.2*pi)*0.9,cos(0:0.1:2.2*pi)*0.9);
      | 
      | % In/out
      | plot([-1.1 -0.9],[0 0]);
      | plot([1.1 0.9],[0 0]);
      | 
      | % 'M'
      | plot([0.5 0.5],[-0.5 0.5]);
      | plot([-0.5 -0.5],[-0.5 0.5]);
      | plot([0.5 0],[0.5 -0.5]);
      | plot([-0.5 0],[0.5 -0.5]);
      | 
      | % Inputs and Outputs
      | plot([0.5 0.5],[0.9 1.8]);
      | plot([0.5 1.1],[1.8 1.8]);
      | 
      | plot([-0.5 -0.5],[0.9 1.8]);
      | plot([-0.5 -1.1],[1.8 1.8]);
      | 
      | 
      | % Plot points to set plot range
      | color('white');plot(1.9,2.8);plot(-1.9,0)
      | color('black');
  Electric Drive3 : Subsystem  Tag=PublishSubsystem
      mask Display:
      | % Circle
      | plot(sin(0:0.1:2.2*pi)*0.9,cos(0:0.1:2.2*pi)*0.9);
      | 
      | % In/out
      | plot([-1.1 -0.9],[0 0]);
      | plot([1.1 0.9],[0 0]);
      | 
      | % 'M'
      | plot([0.5 0.5],[-0.5 0.5]);
      | plot([-0.5 -0.5],[-0.5 0.5]);
      | plot([0.5 0],[0.5 -0.5]);
      | plot([-0.5 0],[0.5 -0.5]);
      | 
      | % Inputs and Outputs
      | plot([0.5 0.5],[0.9 1.8]);
      | plot([0.5 1.1],[1.8 1.8]);
      | 
      | plot([-0.5 -0.5],[0.9 1.8]);
      | plot([-0.5 -1.1],[1.8 1.8]);
      | 
      | 
      | % Plot points to set plot range
      | color('white');plot(1.9,2.8);plot(-1.9,0)
      | color('black');
  Electrical Measurements : Subsystem  Commented=on
  Electrical Reference : fl_lib/Electrical/Electrical Elements/Electrical Reference
  From1 : From  Commented=on  GotoTag=Mot_RPM_SYS_2  TagVisibility=global
  From2 : From  Commented=on  GotoTag=Batt_SYS  TagVisibility=global
  From3 : From  Commented=on  GotoTag=Mot_RPM_SYS_1  TagVisibility=global
  From4 : From  Commented=on  GotoTag=DCDC_SYS
  From5 : From  Commented=on  GotoTag=Mot_RPM_SYS_3  TagVisibility=global
  From6 : From  Commented=on  GotoTag=Mot_RPM_SYS_4  TagVisibility=global
  Goto1 : Goto  Commented=on  GotoTag=Batt_SYS  TagVisibility=global
  Solver Configuration : nesl_utility/Solver Configuration  PhysicalDomain=network_engine_domain  SubClassName=solver  LeftPortType=input  RightPortType=generic  Tones=[]  Harmonics=[]  SimulateNoise=off  Profile=off  UseLocalSampling=off  EnableSwitchedLinearOptims=on  FrequencyDomain=off  UseCCode=off  RelTol=0.001  AbsTol=0.001  MinStep=1e-09  ToWorkspace=off  RevertToSquareIcSolve=off  NumHomotopyIterations=100  PhasorMode=off  PhasorModeNumHarmonics=1  ConsistencySolver=NEWTON_XTOL_AFTER_FTOL  IndexReductionMethod=DerivativeReplacement  DoDC=off  ResidualTolerance=1e-09  ConsistencyTolSource=GLOBAL  ConsistencyAbsTol=0.001  ConsistencyRelTol=0.001  ConsistencyTolFactor=0.001  UseLocalSolver=off  LocalSolverChoice=NE_BACKWARD_EULER_ADVANCER  ResolveIndetEquations=on  FunctionEvalNumThread=1  LocalSolverSampleTime=0.001  DoFixedCost=off  MaxNonlinIter=3  MaxModeIter=2  ComputeImpulses=off  ImpulseIterations=2  LinearAlgebra=auto  LinearAlgebraNumThread=0  EquationFormulation=NE_TIME_EF  DelaysMemoryBudget=1024  AutomaticFiltering=on  FilteringTimeConstant=0.001  PartitionStorageMethod=AS_NEEDED  PartitionMemoryBudget=1024  PartitionMethod=ROBUST  MultibodyUseLocalSolver=off  MultibodyLocalSolverChoice=ODE1  MultibodyLocalSolverSampleTime=0.001
  Speed Sensor5 : Subsystem
      mask Display: disp('S');
  Speed Sensor6 : Subsystem
      mask Display: disp('S');
  Speed Sensor7 : Subsystem
      mask Display: disp('S');
  Speed Sensor8 : Subsystem
      mask Display: disp('S');
  ESys : Outport  VectorParamsAs1DForOutWhenUnconnected=off
  wires:
  From2/1 -> Bus Creator/1
  Bus Creator/1 -> ESys/1
  Battery/1 -> Goto1/1  "Batt"
  From3/1 -> Bus Creator/2
  Mot_TReq1/1 -> Drive Controller1/1(trqR)
  Mot_TReq3/1 -> Drive Controller3/1(trqR)
  From1/1 -> Bus Creator/3
  From5/1 -> Bus Creator/4
  From6/1 -> Bus Creator/5
  From4/1 -> Bus Creator/6
  Drive Controller/2(VdqRef) -> Electric Drive/1(VdqRef)
  Electric Drive/1(M) -> Drive Controller/2(M)
  Mot_TReq/1 -> Drive Controller/1(trqR)
  Drive Controller1/2(VdqRef) -> Electric Drive1/1(VdqRef)
  Electric Drive1/1(M) -> Drive Controller1/2(M)
  Electric Drive2/1(M) -> Drive Controller2/2(M)
  Mot_TReq2/1 -> Drive Controller2/1(trqR)
  Drive Controller2/2(VdqRef) -> Electric Drive2/1(VdqRef)
  Drive Controller3/2(VdqRef) -> Electric Drive3/1(VdqRef)
  Electric Drive3/1(M) -> Drive Controller3/2(M)
  connections:
  Electric Drive1/RConn1 -- Electric Drive3/RConn1 -- Electric Drive2/RConn1 -- Battery (Table-Based)/LConn1 -- Electric Drive/RConn1
  Electric Drive1/LConn1 -- Speed Sensor7/LConn1
  Speed Sensor5/LConn1 -- Electric Drive3/LConn1
  Electric Drive2/LConn1 -- Speed Sensor6/LConn1
  Speed Sensor8/LConn1 -- Electric Drive/LConn1
  Electrical Reference/LConn1 -- Solver Configuration/RConn1 -- Battery (Table-Based)/RConn1

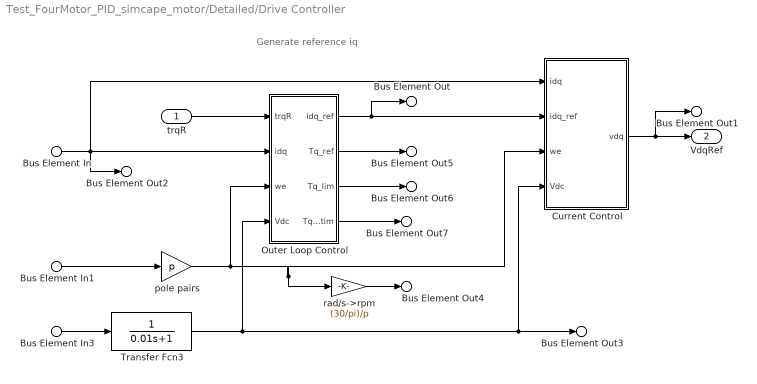
== system Test_FourMotor_PID_simcape_motor/Detailed/Drive Controller ==
  note: Generate reference iq
  trqR : Inport
  Bus Element In : Inport  Port=2  PortName=M  Element=idq
  Bus Element In1 : Inport  Port=2  PortName=M  Element=w
  Bus Element In3 : Inport  Port=2  PortName=M  Element=vdc
  Current Control : Subsystem
  Outer Loop Control : Subsystem
  Transfer Fcn3 : TransferFcn  Denominator=[0.01 1]
  pole pairs : Gain  Gain=p
  rad/s->rpm : Gain  Gain=(30/pi)/p
  Bus Element Out : Outport  PortName=EM  Element=idqRef
  Bus Element Out1 : Outport  PortName=EM  Element=vdq
  Bus Element Out2 : Outport  PortName=EM  Element=idq
  Bus Element Out3 : Outport  PortName=EM  Element=vdc
  Bus Element Out4 : Outport  PortName=EM  Element=rpm
  Bus Element Out5 : Outport  PortName=EM  Element=trqR
  Bus Element Out6 : Outport  PortName=EM  Element=trqLim
  Bus Element Out7 : Outport  PortName=EM  Element=trqEst
  VdqRef : Outport  Port=2  VectorParamsAs1DForOutWhenUnconnected=off
  wires:
  Outer Loop Control/2(Tq_ref) -> Bus Element Out5/1
  Bus Element In/1 -> Bus Element Out2/1, Outer Loop Control/2(idq), Current Control/1(idq)
  Outer Loop Control/3(Tq_lim) -> Bus Element Out6/1
  Transfer Fcn3/1 -> Bus Element Out3/1, Current Control/4(Vdc), Outer Loop Control/4(Vdc)
  Outer Loop Control/1(idq_ref) -> Current Control/2(idq_ref), Bus Element Out/1
  pole pairs/1 -> rad/s->rpm/1, Current Control/3(we), Outer Loop Control/3(we)
  rad/s->rpm/1 -> Bus Element Out4/1
  trqR/1 -> Outer Loop Control/1(trqR)
  Current Control/1(vdq) -> VdqRef/1, Bus Element Out1/1
  Bus Element In3/1 -> Transfer Fcn3/1
  Bus Element In1/1 -> pole pairs/1
  Outer Loop Control/4(Tq_estim) -> Bus Element Out7/1

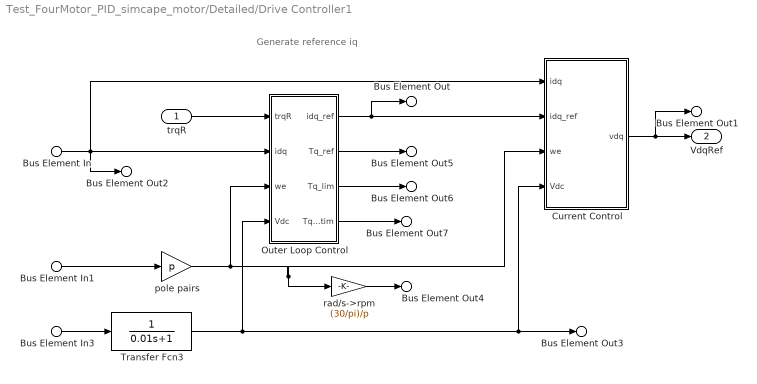
== system Test_FourMotor_PID_simcape_motor/Detailed/Drive Controller1 ==
  note: Generate reference iq
  trqR : Inport
  Bus Element In : Inport  Port=2  PortName=M  Element=idq
  Bus Element In1 : Inport  Port=2  PortName=M  Element=w
  Bus Element In3 : Inport  Port=2  PortName=M  Element=vdc
  Current Control : Subsystem
  Outer Loop Control : Subsystem
  Transfer Fcn3 : TransferFcn  Denominator=[0.01 1]
  pole pairs : Gain  Gain=p
  rad/s->rpm : Gain  Gain=(30/pi)/p
  Bus Element Out : Outport  PortName=EM  Element=idqRef
  Bus Element Out1 : Outport  PortName=EM  Element=vdq
  Bus Element Out2 : Outport  PortName=EM  Element=idq
  Bus Element Out3 : Outport  PortName=EM  Element=vdc
  Bus Element Out4 : Outport  PortName=EM  Element=rpm
  Bus Element Out5 : Outport  PortName=EM  Element=trqR
  Bus Element Out6 : Outport  PortName=EM  Element=trqLim
  Bus Element Out7 : Outport  PortName=EM  Element=trqEst
  VdqRef : Outport  Port=2  VectorParamsAs1DForOutWhenUnconnected=off
  wires:
  Outer Loop Control/2(Tq_ref) -> Bus Element Out5/1
  Bus Element In/1 -> Bus Element Out2/1, Outer Loop Control/2(idq), Current Control/1(idq)
  Outer Loop Control/3(Tq_lim) -> Bus Element Out6/1
  Transfer Fcn3/1 -> Bus Element Out3/1, Current Control/4(Vdc), Outer Loop Control/4(Vdc)
  Outer Loop Control/1(idq_ref) -> Current Control/2(idq_ref), Bus Element Out/1
  pole pairs/1 -> rad/s->rpm/1, Current Control/3(we), Outer Loop Control/3(we)
  rad/s->rpm/1 -> Bus Element Out4/1
  trqR/1 -> Outer Loop Control/1(trqR)
  Current Control/1(vdq) -> VdqRef/1, Bus Element Out1/1
  Bus Element In3/1 -> Transfer Fcn3/1
  Bus Element In1/1 -> pole pairs/1
  Outer Loop Control/4(Tq_estim) -> Bus Element Out7/1

== system Test_FourMotor_PID_simcape_motor/Detailed/Drive Controller2 ==
  note: Generate reference iq
  trqR : Inport
  Bus Element In : Inport  Port=2  PortName=M  Element=idq
  Bus Element In1 : Inport  Port=2  PortName=M  Element=w
  Bus Element In3 : Inport  Port=2  PortName=M  Element=vdc
  Current Control : Subsystem
  Outer Loop Control : Subsystem
  Transfer Fcn3 : TransferFcn  Denominator=[0.01 1]
  pole pairs : Gain  Gain=p
  rad/s->rpm : Gain  Gain=(30/pi)/p
  Bus Element Out : Outport  PortName=EM  Element=idqRef
  Bus Element Out1 : Outport  PortName=EM  Element=vdq
  Bus Element Out2 : Outport  PortName=EM  Element=idq
  Bus Element Out3 : Outport  PortName=EM  Element=vdc
  Bus Element Out4 : Outport  PortName=EM  Element=rpm
  Bus Element Out5 : Outport  PortName=EM  Element=trqR
  Bus Element Out6 : Outport  PortName=EM  Element=trqLim
  Bus Element Out7 : Outport  PortName=EM  Element=trqEst
  VdqRef : Outport  Port=2  VectorParamsAs1DForOutWhenUnconnected=off
  wires:
  Outer Loop Control/2(Tq_ref) -> Bus Element Out5/1
  Bus Element In/1 -> Bus Element Out2/1, Outer Loop Control/2(idq), Current Control/1(idq)
  Outer Loop Control/3(Tq_lim) -> Bus Element Out6/1
  Transfer Fcn3/1 -> Bus Element Out3/1, Current Control/4(Vdc), Outer Loop Control/4(Vdc)
  Outer Loop Control/1(idq_ref) -> Current Control/2(idq_ref), Bus Element Out/1
  pole pairs/1 -> rad/s->rpm/1, Current Control/3(we), Outer Loop Control/3(we)
  rad/s->rpm/1 -> Bus Element Out4/1
  trqR/1 -> Outer Loop Control/1(trqR)
  Current Control/1(vdq) -> VdqRef/1, Bus Element Out1/1
  Bus Element In3/1 -> Transfer Fcn3/1
  Bus Element In1/1 -> pole pairs/1
  Outer Loop Control/4(Tq_estim) -> Bus Element Out7/1

== system Test_FourMotor_PID_simcape_motor/Detailed/Drive Controller3 ==
  note: Generate reference iq
  trqR : Inport
  Bus Element In : Inport  Port=2  PortName=M  Element=idq
  Bus Element In1 : Inport  Port=2  PortName=M  Element=w
  Bus Element In3 : Inport  Port=2  PortName=M  Element=vdc
  Current Control : Subsystem
  Outer Loop Control : Subsystem
  Transfer Fcn3 : TransferFcn  Denominator=[0.01 1]
  pole pairs : Gain  Gain=p
  rad/s->rpm : Gain  Gain=(30/pi)/p
  Bus Element Out : Outport  PortName=EM  Element=idqRef
  Bus Element Out1 : Outport  PortName=EM  Element=vdq
  Bus Element Out2 : Outport  PortName=EM  Element=idq
  Bus Element Out3 : Outport  PortName=EM  Element=vdc
  Bus Element Out4 : Outport  PortName=EM  Element=rpm
  Bus Element Out5 : Outport  PortName=EM  Element=trqR
  Bus Element Out6 : Outport  PortName=EM  Element=trqLim
  Bus Element Out7 : Outport  PortName=EM  Element=trqEst
  VdqRef : Outport  Port=2  VectorParamsAs1DForOutWhenUnconnected=off
  wires:
  Outer Loop Control/2(Tq_ref) -> Bus Element Out5/1
  Bus Element In/1 -> Bus Element Out2/1, Outer Loop Control/2(idq), Current Control/1(idq)
  Outer Loop Control/3(Tq_lim) -> Bus Element Out6/1
  Transfer Fcn3/1 -> Bus Element Out3/1, Current Control/4(Vdc), Outer Loop Control/4(Vdc)
  Outer Loop Control/1(idq_ref) -> Current Control/2(idq_ref), Bus Element Out/1
  pole pairs/1 -> rad/s->rpm/1, Current Control/3(we), Outer Loop Control/3(we)
  rad/s->rpm/1 -> Bus Element Out4/1
  trqR/1 -> Outer Loop Control/1(trqR)
  Current Control/1(vdq) -> VdqRef/1, Bus Element Out1/1
  Bus Element In3/1 -> Transfer Fcn3/1
  Bus Element In1/1 -> pole pairs/1
  Outer Loop Control/4(Tq_estim) -> Bus Element Out7/1
